simulink model "PID_Simulink"  (R2019b)
settings: Solver=FixedStepAuto  StartTime=0.0  StopTime=10.0  FixedStep=0.0001  RelTol=1e-3
values from neighbouring files (symbols this model uses):
  B = (NL_current*Km)/NL_speed    (= 7.06678023853e-07)    [DCX19_Motor_Calculations.m]
  desired_angle_vectors = [pi/2 -1.57 1.57/2]    [DCX19_Motor_Calculations.m]
  J = 2.72*10^-7    (= 2.72e-07)    [DCX19_Motor_Calculations.m]
  Kb = 1/(268*(2*pi/60))    (= 0.0356317036773)    [DCX19_Motor_Calculations.m]
  Km = 35.6*10^-3    (= 0.0356)    [DCX19_Motor_Calculations.m]
  L = 1.320*10^-3    (= 0.00132)    [DCX19_Motor_Calculations.m]
  res = (2*pi)/CPR    (= 0.0490873852123)    [DCX19_Motor_Calculations.m]
undefined symbols (not defined in the file or in its folder): R
libraries: cstblocks x3
settings Model: Creator=harsh  LastModifiedBy=harsh

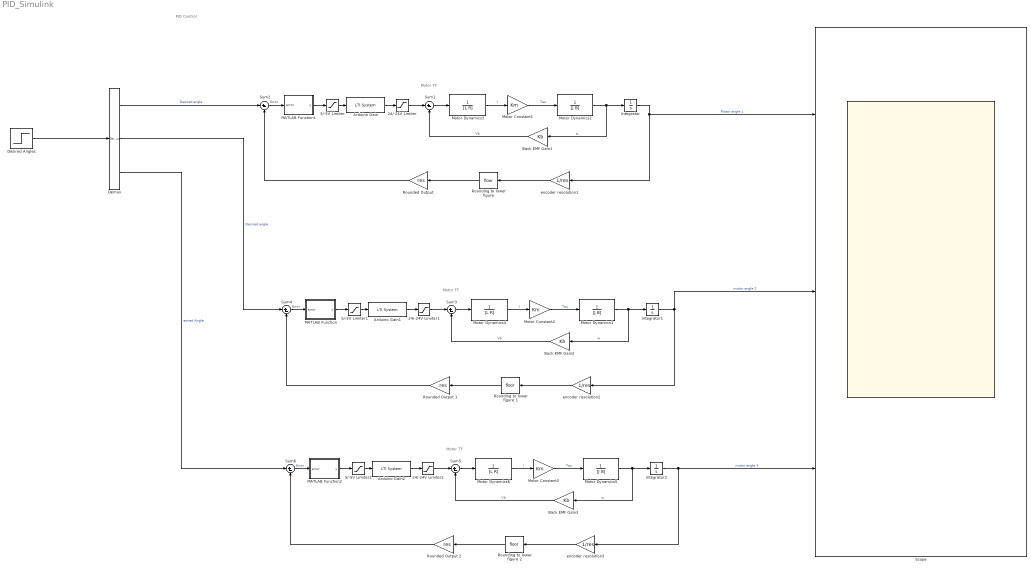
== system PID_Simulink ==
  note: PID Control
  note: Motor TF
  note: Motor TF
  note: Motor TF
  24/-24V Limiter : Saturate  UpperLimit=5  LowerLimit=-5
  24/-24V Limiter1 : Saturate  UpperLimit=5  LowerLimit=-5
  24/-24V Limiter2 : Saturate  UpperLimit=5  LowerLimit=-5
  5/-5V Limiter : Saturate  UpperLimit=5  LowerLimit=-5
  5/-5V Limiter1 : Saturate  UpperLimit=5  LowerLimit=-5
  5/-5V Limiter2 : Saturate  UpperLimit=5  LowerLimit=-5
  Arduino Gain : cstblocks/LTI System  sys=OPAMP  IC=[]
  Arduino Gain1 : cstblocks/LTI System  sys=OPAMP  IC=[]
  Arduino Gain2 : cstblocks/LTI System  sys=OPAMP  IC=[]
  Back EMF Gain1 : Gain  Gain=Kb
  Back EMF Gain2 : Gain  Gain=Kb
  Back EMF Gain3 : Gain  Gain=Kb
  Demux : Demux  Outputs=3
  "Desired Angles " : Step  After=desired_angle_vectors  SampleTime=0
  Integrator : Integrator
  Integrator1 : Integrator
  Integrator2 : Integrator
  MATLAB Function : MATLAB Function  TreatAsAtomicUnit=on
  MATLAB Function1 : MATLAB Function  TreatAsAtomicUnit=on
  MATLAB Function2 : MATLAB Function  TreatAsAtomicUnit=on
  Motor Constant1 : Gain  Gain=Km
  Motor Constant2 : Gain  Gain=Km
  Motor Constant3 : Gain  Gain=Km
  Motor Dynamics1 : TransferFcn  Denominator=[J B]
  Motor Dynamics2 : TransferFcn  Denominator=[J B]
  Motor Dynamics3 : TransferFcn  Denominator=[L R]
  Motor Dynamics4 : TransferFcn  Denominator=[L R]
  Motor Dynamics5 : TransferFcn  Denominator=[J B]
  Motor Dynamics6 : TransferFcn  Denominator=[L R]
  "Rounded Output " : Gain  Gain=res
  Rounded Output 1 : Gain  Gain=res
  Rounded Output 2 : Gain  Gain=res
  "Rounding to lower figure " : Rounding
  Rounding to lower figure 1 : Rounding
  Rounding to lower figure 2 : Rounding
  Scope : Scope  NumInputPorts=3
  Sum{1..6} (6 alike) : Sum  Inputs=|+-
  encoder resolution1 : Gain  Gain=1/res
  encoder resolution2 : Gain  Gain=1/res
  encoder resolution3 : Gain  Gain=1/res
  wires:
  "Desired Angles "/1 -> Demux/1
  Demux/2 -> Sum4/1  "Desired angle"
  Back EMF Gain1/1 -> Sum1/2  "Vb"
  Sum2/1 -> MATLAB Function1/1(error)  "Error"
  Motor Dynamics2/1 -> Integrator/1, Back EMF Gain1/1  "w"
  5/-5V Limiter/1 -> Arduino Gain/1
  Integrator/1 -> Scope/1, encoder resolution1/1  "Motor angle 1"
  24/-24V Limiter/1 -> Sum1/1
  Motor Dynamics3/1 -> Motor Constant1/1  "I"
  Sum1/1 -> Motor Dynamics3/1
  Arduino Gain/1 -> 24/-24V Limiter/1
  Motor Constant1/1 -> Motor Dynamics2/1  "Tau"
  "Rounding to lower figure "/1 -> "Rounded Output "/1
  MATLAB Function1/1(y) -> 5/-5V Limiter/1
  "Rounded Output "/1 -> Sum2/2
  encoder resolution1/1 -> "Rounding to lower figure "/1
  Demux/1 -> Sum2/1  "Desired angle"
  Back EMF Gain2/1 -> Sum3/2  "Vb"
  Sum4/1 -> MATLAB Function/1(error)  "Error"
  Motor Dynamics1/1 -> Integrator1/1, Back EMF Gain2/1  "w"
  5/-5V Limiter1/1 -> Arduino Gain1/1
  Integrator1/1 -> Scope/2, encoder resolution2/1  "motor angle 2"
  24/-24V Limiter1/1 -> Sum3/1
  Motor Dynamics4/1 -> Motor Constant2/1  "I"
  Sum3/1 -> Motor Dynamics4/1
  Arduino Gain1/1 -> 24/-24V Limiter1/1
  Motor Constant2/1 -> Motor Dynamics1/1  "Tau"
  Rounding to lower figure 1/1 -> Rounded Output 1/1
  MATLAB Function/1(y) -> 5/-5V Limiter1/1
  Rounded Output 1/1 -> Sum4/2
  encoder resolution2/1 -> Rounding to lower figure 1/1
  Back EMF Gain3/1 -> Sum5/2  "Vb"
  Sum6/1 -> MATLAB Function2/1(error)  "Error"
  Motor Dynamics5/1 -> Integrator2/1, Back EMF Gain3/1  "w"
  5/-5V Limiter2/1 -> Arduino Gain2/1
  Integrator2/1 -> Scope/3, encoder resolution3/1  "motor angle 3"
  24/-24V Limiter2/1 -> Sum5/1
  Motor Dynamics6/1 -> Motor Constant3/1  "I"
  Sum5/1 -> Motor Dynamics6/1
  Arduino Gain2/1 -> 24/-24V Limiter2/1
  Motor Constant3/1 -> Motor Dynamics5/1  "Tau"
  Rounding to lower figure 2/1 -> Rounded Output 2/1
  MATLAB Function2/1(y) -> 5/-5V Limiter2/1
  Rounded Output 2/1 -> Sum6/2
  encoder resolution3/1 -> Rounding to lower figure 2/1
  Demux/3 -> Sum6/1  "esired Angle"

== matlab function PID_Simulink/MATLAB Function1 ==
  settings: updateMethod=DISCRETE
  data: error input; y output
function y = fcn(error)

persistent previous_error;                  %previous error = current error for next iteration, initially set to 0;
persistent Ki_output;                        %need as persistent variable for Ki_output = Ki_output + (...)
persistent ept;                             %constant vector of exponentials (p*e^(-p*n*Ts)) where n = 1.....#of samples we want to average
persistent unweighted_differential_outputs;  %vector used for dot product with ept, shifted at each cycle. 

if isempty(previous_error)
    previous_error = 0;
end

%Trial values for testing against Built in PID block
Kp = 0.223809;
Ki = 0.111836;
Kd = 0.012272;

Ts = 0.0001;    %Controller frequency from Arduino assumed to be 10kHz.

%--------P controller part------------------
Kp_output = Kp*error;    

%---------I controller part-----------------

%Initializing Ki_output
if isempty(Ki_output)
    Ki_output = 0;
end

Ki_output = Ki_output + Ki*[(error + previous_error)/2]*Ts; %cumulative areas of trapeziums

%----------D controller part----------------
controlfreq = 10000; %Hz
filter_pole = 4000;  %big pole because we don't care much about averaging but we do care a lot about delay. (signal is not noisy)
n = 4*controlfreq/filter_pole;  %We are averaging 80 samples in this example


%Now, we initialize the ept vector (will remain constant valued throughout the program)
if isempty(ept)
    ept = zeros(1,n);
    for i = 1:n
        ept(i) = filter_pole*1.132*exp(-filter_pole*i*Ts);
    end
    %We want Ts*sum(ept) = 1 but this is not the case normally, so we have to scale the ept such that we get a sum
    %of 1. To account for discretization error, we scale it by multiplying it by 1.132 in this example. 
end

if isempty(unweighted_differential_outputs)
    unweighted_differential_outputs = zeros(1,n);
end 

unweighted_differential_outputs(1) = (error - previous_error); 
filtered_derivative = dot(ept,unweighted_differential_outputs);

Kd_output = Kd*filtered_derivative;

n2 = n+1; %n2 = 9
for count = 1:(n-1) %1:7 in this example
    unweighted_differential_outputs(n2-count) = unweighted_differential_outputs(n2 - count - 1);    %shift values by one index, and in next loop calculate one more new slope at index 1 (starting index)
end 

y = Kp_output + Ki_output + Kd_output;

previous_error = error; %this will help us move on to get new values for Ki and Kd

end

== matlab function PID_Simulink/MATLAB Function ==
  settings: updateMethod=DISCRETE
  data: error input; y output
function y = fcn(error)

persistent previous_error;                  %previous error = current error for next iteration, initially set to 0;
persistent Ki_output;                        %need as persistent variable for Ki_output = Ki_output + (...)
persistent ept;                             %constant vector of exponentials (p*e^(-p*n*Ts)) where n = 1.....#of samples we want to average
persistent unweighted_differential_outputs;  %vector used for dot product with ept, shifted at each cycle. 

if isempty(previous_error)
    previous_error = 0;
end

%Trial values for testing against Built in PID block
Kp = 0.223809;
Ki = 0.111836;
Kd = 0.012272;

Ts = 0.0001;    %Controller frequency from Arduino assumed to be 10kHz.

%--------P controller part------------------
Kp_output = Kp*error;    

%---------I controller part-----------------

%Initializing Ki_output
if isempty(Ki_output)
    Ki_output = 0;
end

Ki_output = Ki_output + Ki*[(error + previous_error)/2]*Ts; %cumulative areas of trapeziums

%----------D controller part----------------
controlfreq = 10000; %Hz
filter_pole = 4000;  %big pole because we don't care much about averaging but we do care a lot about delay. (signal is not noisy)
n = 4*controlfreq/filter_pole;  %We are averaging 80 samples in this example


%Now, we initialize the ept vector (will remain constant valued throughout the program)
if isempty(ept)
    ept = zeros(1,n);
    for i = 1:n
        ept(i) = filter_pole*1.132*exp(-filter_pole*i*Ts);
    end
    %We want Ts*sum(ept) = 1 but this is not the case normally, so we have to scale the ept such that we get a sum
    %of 1. To account for discretization error, we scale it by multiplying it by 1.132 in this example. 
end

if isempty(unweighted_differential_outputs)
    unweighted_differential_outputs = zeros(1,n);
end 

unweighted_differential_outputs(1) = (error - previous_error); 
filtered_derivative = dot(ept,unweighted_differential_outputs);

Kd_output = Kd*filtered_derivative;

n2 = n+1; %n2 = 9
for count = 1:(n-1) %1:7 in this example
    unweighted_differential_outputs(n2-count) = unweighted_differential_outputs(n2 - count - 1);    %shift values by one index, and in next loop calculate one more new slope at index 1 (starting index)
end 

y = Kp_output + Ki_output + Kd_output;

previous_error = error; %this will help us move on to get new values for Ki and Kd

end

== matlab function PID_Simulink/MATLAB Function2 ==
  settings: updateMethod=DISCRETE
  data: error input; y output
function y = fcn(error)

persistent previous_error;                  %previous error = current error for next iteration, initially set to 0;
persistent Ki_output;                        %need as persistent variable for Ki_output = Ki_output + (...)
persistent ept;                             %constant vector of exponentials (p*e^(-p*n*Ts)) where n = 1.....#of samples we want to average
persistent unweighted_differential_outputs;  %vector used for dot product with ept, shifted at each cycle. 

if isempty(previous_error)
    previous_error = 0;
end

%Trial values for testing against Built in PID block
Kp = 0.223809;
Ki = 0.111836;
Kd = 0.012272;

Ts = 0.0001;    %Controller frequency from Arduino assumed to be 10kHz.

%--------P controller part------------------
Kp_output = Kp*error;    

%---------I controller part-----------------

%Initializing Ki_output
if isempty(Ki_output)
    Ki_output = 0;
end

Ki_output = Ki_output + Ki*[(error + previous_error)/2]*Ts; %cumulative areas of trapeziums

%----------D controller part----------------
controlfreq = 10000; %Hz
filter_pole = 4000;  %big pole because we don't care much about averaging but we do care a lot about delay. (signal is not noisy)
n = 4*controlfreq/filter_pole;  %We are averaging 80 samples in this example


%Now, we initialize the ept vector (will remain constant valued throughout the program)
if isempty(ept)
    ept = zeros(1,n);
    for i = 1:n
        ept(i) = filter_pole*1.132*exp(-filter_pole*i*Ts);
    end
    %We want Ts*sum(ept) = 1 but this is not the case normally, so we have to scale the ept such that we get a sum
    %of 1. To account for discretization error, we scale it by multiplying it by 1.132 in this example. 
end

if isempty(unweighted_differential_outputs)
    unweighted_differential_outputs = zeros(1,n);
end 

unweighted_differential_outputs(1) = (error - previous_error); 
filtered_derivative = dot(ept,unweighted_differential_outputs);

Kd_output = Kd*filtered_derivative;

n2 = n+1; %n2 = 9
for count = 1:(n-1) %1:7 in this example
    unweighted_differential_outputs(n2-count) = unweighted_differential_outputs(n2 - count - 1);    %shift values by one index, and in next loop calculate one more new slope at index 1 (starting index)
end 

y = Kp_output + Ki_output + Kd_output;

previous_error = error; %this will help us move on to get new values for Ki and Kd

end
